simulink model "nanodrum"  (R2018a)
settings: Solver=VariableStepAuto  StartTime=0.0  StopTime=6/f  MaxStep=1/f/1000  RelTol=1e-3  EnableMultiTasking=on
model workspace (MAT data in the model file):
  C = 1e-06
  R = 50
  V = 0.001
  f = 2000
  gm1 = 0.143634273378
  gm2 = 0.02
  ph = 0.174532925199
  w = 12566.3706144
libraries: fl_lib x23, nesl_utility x3
CloseFcn:
  | try,close(nanodrum_frequency_response),end
  | clear nanodrum_frequency_response
  | try,close(nanodrum_frequency_response),end
  | clear nanodrum_frequency_response
  | 
  | clear simlog_nanodrum
  | clear logsout_nanodrum
Description:
  | Porous Graphene Nanodrum
  | 
  | Copyright Irek Roslon 2018
settings Model: Creator=IrekRoslon  LastModifiedBy=Irek
settings DataIOCC: MaxDataPoints=15000  SaveOutput=off  DSMLogging=off  SaveTime=off  SignalLoggingName=logsout_elec_filter_phase_ota
settings OptimizationCC: ExpressionDepthLimit=2147483647  LifeSpan=inf
settings DebuggingCC: UnderspecifiedInitializationDetection=Classic  MergeDetectMultiDrivingBlocksExec=none  SolverPrmCheckMsg=warning  FcnCallInpInsideContextMsg=warning  StateNameClashWarn=warning  SFUnexpectedBacktrackingDiag=warning  SFNoUnconditionalDefaultTransitionDiag=warning  SFExecutionAtInitializationDiag=none
settings HardwareCC: ProdBitPerPointer=32  ProdBitPerSizeT=32  ProdBitPerPtrDiffT=32  ProdLargestAtomicFloat=None  ProdIntDivRoundTo=Undefined  ProdEndianess=Unspecified  ProdWordSize=32  ProdHWDeviceType=32-bit Generic
settings ModelReferenceCC: PropagateSignalLabelsOutOfModel=off
settings CodeAppCC: StateflowObjectComments=on
settings GRTTargetCC: TargetLangStandard=C89/C90 (ANSI)  GeneratePreprocessorConditionals=Disable all  CombineOutputUpdateFcns=off  GRTInterface=on
settings ConfigComp: CovMetricSettings=dw  CovHtmlReporting=on  CovSaveCumulativeToWorkspaceVar=on  CovSaveSingleToWorkspaceVar=on  CovExternalEMLEnable=off  CovSFcnEnable=off
settings SimscapeCC: SimscapeLogType=all  SimscapeLogSimulationStatistics=on  SimscapeLogName=simlog_elec_filter_phase_ota  SimscapeLogDataHistory=15000

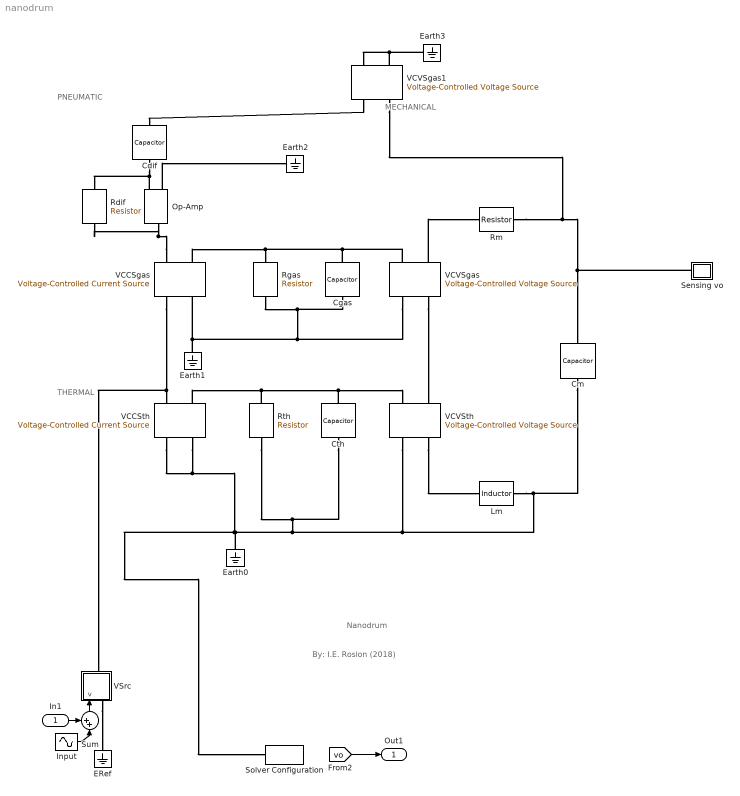
== system nanodrum ==
  note: Nanodrum
  note: THERMAL
  note: PNEUMATIC
  note: MECHANICAL
  note: By: I.E. Roslon (2018)
  In1 : Inport
  Cdif : fl_lib/Electrical/Electrical Elements/Capacitor  c=1 F  r=1e-22 Ohm  g=0 1/Ohm  i_specify=off  i_priority=None  i=0 A  i_nominal_specify=off  i_nominal_unit=A  i_nominal_value=1  v_specify=off  v_priority=None  v=0 V  v_nominal_specify=off  v_nominal_unit=V  v_nominal_value=1  vc_specify=off  vc_priority=High  vc=0 V  vc_nominal_specify=off  vc_nominal_unit=V  vc_nominal_value=1
  Cgas : fl_lib/Electrical/Electrical Elements/Capacitor  c=8.5e-22 F  r=1e-25 Ohm  g=0 1/Ohm  i_specify=off  i_priority=None  i=0 A  i_nominal_specify=off  i_nominal_unit=A  i_nominal_value=1  v_specify=off  v_priority=None  v=0 V  v_nominal_specify=off  v_nominal_unit=V  v_nominal_value=1  vc_specify=off  vc_priority=High  vc=0 V  vc_nominal_specify=off  vc_nominal_unit=V  vc_nominal_value=1
  Cm : fl_lib/Electrical/Electrical Elements/Capacitor  c=0.0037 F  r=1e-10 Ohm  g=0 1/Ohm  i_specify=off  i_priority=None  i=0 A  i_nominal_specify=off  i_nominal_unit=A  i_nominal_value=1  v_specify=off  v_priority=None  v=0 V  v_nominal_specify=off  v_nominal_unit=V  v_nominal_value=1  vc_specify=off  vc_priority=High  vc=0 V  vc_nominal_specify=off  vc_nominal_unit=V  vc_nominal_value=1
  Cth : fl_lib/Electrical/Electrical Elements/Capacitor  c=2.65e-15 F  r=1e-22 Ohm  g=0 1/Ohm  i_specify=off  i_priority=None  i=0 A  i_nominal_specify=off  i_nominal_unit=A  i_nominal_value=1  v_specify=off  v_priority=None  v=0 V  v_nominal_specify=off  v_nominal_unit=V  v_nominal_value=1  vc_specify=off  vc_priority=High  vc=0 V  vc_nominal_specify=off  vc_nominal_unit=V  vc_nominal_value=1
  ERef : fl_lib/Electrical/Electrical Elements/Electrical Reference
      settings: SourceProductName=Foundation Library
  Earth{0..3} (4 alike) : fl_lib/Electrical/Electrical Elements/Electrical Reference
  Input : Sin  Amplitude=V  Frequency=2*pi*f  SampleTime=0
  Lm : fl_lib/Electrical/Electrical Elements/Inductor  l=5.5e-15 H  r=0 Ohm  g=0 1/Ohm  i_specify=off  i_priority=None  i=0 A  i_nominal_specify=off  i_nominal_unit=A  i_nominal_value=1  v_specify=off  v_priority=None  v=0 V  v_nominal_specify=off  v_nominal_unit=V  v_nominal_value=1  i_L_specify=off  i_L_priority=High  i_L=0 A  i_L_nominal_specify=off  i_L_nominal_unit=A  i_L_nominal_value=1
  Op-Amp : fl_lib/Electrical/Electrical Elements/Op-Amp  outI_specify=off  outI_priority=None  outI=0 A  outI_nominal_specify=off  outI_nominal_unit=A  outI_nominal_value=1
  Rdif : fl_lib/Electrical/Electrical Elements/Resistor  R=1 Ohm  i_specify=off  i_priority=None  i=0 A  i_nominal_specify=off  i_nominal_unit=A  i_nominal_value=1  v_specify=off  v_priority=None  v=0 V  v_nominal_specify=off  v_nominal_unit=V  v_nominal_value=1
  Rgas : fl_lib/Electrical/Electrical Elements/Resistor  R=9.43e14 Ohm  i_specify=off  i_priority=None  i=0 A  i_nominal_specify=off  i_nominal_unit=A  i_nominal_value=1  v_specify=off  v_priority=None  v=0 V  v_nominal_specify=off  v_nominal_unit=V  v_nominal_value=1
  Rm : fl_lib/Electrical/Electrical Elements/Resistor  R=1e-8 Ohm  i_specify=off  i_priority=None  i=0 A  i_nominal_specify=off  i_nominal_unit=A  i_nominal_value=1  v_specify=off  v_priority=None  v=0 V  v_nominal_specify=off  v_nominal_unit=V  v_nominal_value=1
  Rth : fl_lib/Electrical/Electrical Elements/Resistor  R=1.32e7 Ohm  i_specify=off  i_priority=None  i=0 A  i_nominal_specify=off  i_nominal_unit=A  i_nominal_value=1  v_specify=off  v_priority=None  v=0 V  v_nominal_specify=off  v_nominal_unit=V  v_nominal_value=1
  Sensing vo : Subsystem
      mask Display: disp('vo');
  Solver Configuration : nesl_utility/Solver Configuration  PhysicalDomain=network_engine_domain  SubClassName=solver  LeftPortType=input  RightPortType=generic  Tones=[]  Harmonics=[]  SimulateNoise=off  Profile=off  UseLocalSampling=off  EnableSwitchedLinearOptims=on  FrequencyDomain=off  UseCCode=off  RelTol=0.001  AbsTol=1e-06  MinStep=1e-09  ToWorkspace=off  RevertToSquareIcSolve=off  NumHomotopyIterations=100  PhasorMode=off  PhasorModeNumHarmonics=1  DoDC=off  ResidualTolerance=1e-9  UseLocalSolver=off  LocalSolverChoice=NE_BACKWARD_EULER_ADVANCER  LocalSolverSampleTime=.001  DoFixedCost=off  MaxNonlinIter=3  MaxModeIter=2  LinearAlgebra=Sparse  EquationFormulation=NE_TIME_EF  DelaysMemoryBudget=1024  AutomaticFiltering=on  FilteringTimeConstant=0.001
  Sum : Sum  Inputs=++|
  VCCSgas : fl_lib/Electrical/Electrical Sources/Voltage-Controlled Current Source  K=-1e-15 1/Ohm  v1_specify=off  v1_priority=None  v1=0 V  v1_nominal_specify=off  v1_nominal_unit=V  v1_nominal_value=1  i2_specify=off  i2_priority=None  i2=0 A  i2_nominal_specify=off  i2_nominal_unit=A  i2_nominal_value=1
      settings: SourceProductName=Simscape  SourceProductBaseCode=SS
  VCCSth : fl_lib/Electrical/Electrical Sources/Voltage-Controlled Current Source  K=-2.65e-8 1/Ohm  v1_specify=off  v1_priority=None  v1=0 V  v1_nominal_specify=off  v1_nominal_unit=V  v1_nominal_value=1  i2_specify=off  i2_priority=None  i2=0 A  i2_nominal_specify=off  i2_nominal_unit=A  i2_nominal_value=1
      settings: SourceProductName=Simscape  SourceProductBaseCode=SS
  VCVSgas : fl_lib/Electrical/Electrical Sources/Voltage-Controlled Voltage Source  K=1  v1_specify=off  v1_priority=None  v1=0 V  v1_nominal_specify=off  v1_nominal_unit=V  v1_nominal_value=1  v2_specify=off  v2_priority=None  v2=0 V  v2_nominal_specify=off  v2_nominal_unit=V  v2_nominal_value=1
      settings: SourceProductName=Simscape  SourceProductBaseCode=SS
  VCVSgas1 : fl_lib/Electrical/Electrical Sources/Voltage-Controlled Voltage Source  K=1e-11  v1_specify=off  v1_priority=None  v1=0 V  v1_nominal_specify=off  v1_nominal_unit=V  v1_nominal_value=1  v2_specify=off  v2_priority=None  v2=0 V  v2_nominal_specify=off  v2_nominal_unit=V  v2_nominal_value=1
      settings: SourceProductName=Simscape  SourceProductBaseCode=SS
  VCVSth : fl_lib/Electrical/Electrical Sources/Voltage-Controlled Voltage Source  K=1  v1_specify=off  v1_priority=None  v1=0 V  v1_nominal_specify=off  v1_nominal_unit=V  v1_nominal_value=1  v2_specify=off  v2_priority=None  v2=0 V  v2_nominal_specify=off  v2_nominal_unit=V  v2_nominal_value=1
      settings: SourceProductName=Simscape  SourceProductBaseCode=SS
  VSrc : Subsystem
  Out1 : Outport
  wires:
  [vo] -> Out1/1
  Sum/1 -> VSrc/1(v)
  Input/1 -> Sum/2
  In1/1 -> Sum/1
  connections:
  VSrc/LConn1 -- ERef/LConn1
  Rth/LConn1 -- Solver Configuration/RConn1 -- VCCSth/RConn1 -- VCCSth/RConn2 -- Earth0/LConn1 -- Lm/RConn1 -- Cm/LConn1 -- VCVSth/RConn1 -- Cth/LConn1
  Rgas/RConn1 -- VCCSgas/LConn2 -- VCVSgas/LConn1 -- Cgas/RConn1
  VCCSth/LConn1 -- VCCSgas/RConn1 -- VSrc/RConn1
  Rm/RConn1 -- VCVSgas1/LConn1 -- Sensing vo/RConn1 -- Cm/RConn1
  VCCSth/LConn2 -- Rth/RConn1 -- Cth/RConn1 -- VCVSth/LConn1
  Earth1/LConn1 -- Rgas/LConn1 -- Cgas/LConn1 -- VCVSgas/RConn1 -- VCCSgas/RConn2
  Cdif/LConn1 -- Op-Amp/LConn2 -- Rdif/LConn1
  VCCSgas/LConn1 -- Op-Amp/RConn1 -- Rdif/RConn1
  Op-Amp/LConn1 -- Earth2/LConn1
  VCVSgas/LConn2 -- Rm/LConn1
  VCVSgas/RConn2 -- VCVSth/LConn2
  VCVSth/RConn2 -- Lm/LConn1
  VCVSgas1/LConn2 -- Cdif/RConn1
  VCVSgas1/RConn1 -- Earth3/LConn1 -- VCVSgas1/RConn2

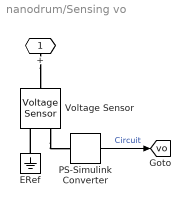
== system nanodrum/Sensing vo ==
  ERef : fl_lib/Electrical/Electrical Elements/Electrical Reference
      settings: SourceProductName=Foundation Library
  PS-Simulink Converter : nesl_utility/PS-Simulink Converter  PhysicalDomain=network_engine_domain  SubClassName=ps_output  LeftPortType=input  RightPortType=output  PseudoPeriodic=off  Frequencies=[]  Unit=V  AffineConversion=off
  Voltage Sensor : fl_lib/Electrical/Electrical Sensors/Voltage Sensor
      settings: SourceProductName=Foundation Library
  + : PMIOPort  Side=Right
  tag scope: vo=global
  wires:
  PS-Simulink Converter/1 -> [vo]  "Circuit"
  connections:
  ERef/LConn1 -- Voltage Sensor/RConn2
  +/RConn1 -- Voltage Sensor/LConn1
  Voltage Sensor/RConn1 -- PS-Simulink Converter/LConn1

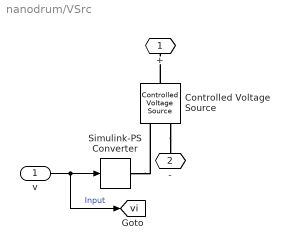
== system nanodrum/VSrc ==
  v : Inport
  Controlled Voltage Source : fl_lib/Electrical/Electrical Sources/Controlled Voltage Source
      settings: SourceProductName=Foundation Library
  Simulink-PS Converter : nesl_utility/Simulink-PS Converter  PhysicalDomain=network_engine_domain  SubClassName=ps_input  LeftPortType=input  RightPortType=output  PseudoPeriodic=off  Frequencies=[]  NoiseDistribution=none  NoiseParameters=[]  Unit=1  AffineConversion=off  FilteringAndDerivatives=zero  SimscapeFilterOrder=1  InputFilterTimeConstant=0.001  UdotUserProvided=1
  + : PMIOPort  Side=Right
  - : PMIOPort  Port=2  Side=Left
  tag scope: vi=global
  wires:
  v/1 -> [vi], Simulink-PS Converter/1  "Input"
  connections:
  Simulink-PS Converter/RConn1 -- Controlled Voltage Source/RConn1
  Controlled Voltage Source/RConn2 -- -/RConn1
  Controlled Voltage Source/LConn1 -- +/RConn1
